simulink model "Gen_stAlone"  (R2018a)
settings: Solver=VariableStepAuto  StartTime=0.0  StopTime=20  MaxStep=1e-3  RelTol=1e-3
libraries: simulink x1
settings Model: Creator=cmparedes  LastModifiedBy=cmparedes

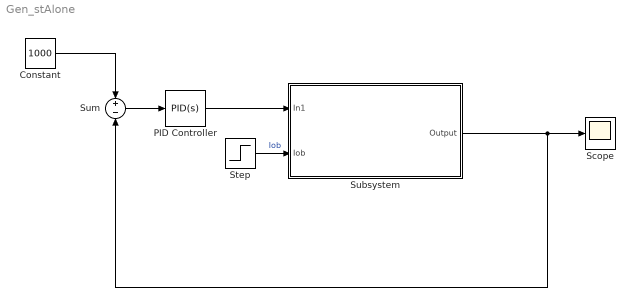
== system Gen_stAlone ==
  Constant : Constant  Value=1000
  PID Controller : simulink/Continuous/PID Controller  Controller=PID  TimeDomain=Continuous-time  SampleTime=-1  IntegratorMethod=Forward Euler  FilterMethod=Forward Euler  Form=Parallel  UseFilter=on  ControllerParametersSource=internal  P=1  I=10  D=0  N=100  InitialConditionSource=internal  InitialConditionForIntegrator=0  InitialConditionForFilter=0  ExternalReset=none  LimitOutput=off  UpperSaturationLimit=inf  LowerSaturationLimit=-inf  LinearizeAsGain=on  AntiWindupMode=none  Kb=1  TrackingMode=off  Kt=1  PParamMin=[]  PParamMax=[]  IParamMin=[]  IParamMax=[]  DParamMin=[]  DParamMax=[]  NParamMin=[]  NParamMax=[]  KbParamMin=[]  KbParamMax=[]  KtParamMin=[]  KtParamMax=[]  POutMin=[]  POutMax=[]  IOutMin=[]  IOutMax=[]  DOutMin=[]  DOutMax=[]  NOutMin=[]  NOutMax=[]  KbOutMin=[]  KbOutMax=[]  KtOutMin=[]  KtOutMax=[]  IntegratorOutMin=[]  IntegratorOutMax=[]  FilterOutMin=[]  FilterOutMax=[]  SumOutMin=[]  SumOutMax=[]  SumI1OutMin=[]  SumI1OutMax=[]  SumI2OutMin=[]  SumI2OutMax=[]  SumI3OutMin=[]  SumI3OutMax=[]  SumDOutMin=[]  SumDOutMax=[]  SaturationOutMin=[]  SaturationOutMax=[]  IntegratorContinuousStateAttributes=''  IntegratorStateMustResolveToSignalObject=off  IntegratorRTWStateStorageClass=Auto  FilterContinuousStateAttributes=''  FilterStateMustResolveToSignalObject=off  FilterRTWStateStorageClass=Auto  DifferentiatorICPrevScaledInput=0  DifferentiatorOutMin=[]  DifferentiatorOutMax=[]  FilterDiffOutCoefMin=[]  FilterDiffOutCoefMax=[]  SumDenOutMin=[]  SumDenOutMax=[]  SumNumOutMin=[]  SumNumOutMax=[]  ReciprocalOutMin=[]  ReciprocalOutMax=[]  DivideOutMin=[]  DivideOutMax=[]  TunerSelectOption=Transfer Function Based (PID Tuner App)
  Scope : Scope
  Step : Step  Time=10  Before=5  After=10  SampleTime=0
  Subsystem : Subsystem
  Sum : Sum  Inputs=+-
  wires:
  Step/1 -> Subsystem/2(Iob)  "Iob"
  Sum/1 -> PID Controller/1
  PID Controller/1 -> Subsystem/1(In1)
  Constant/1 -> Sum/1
  Subsystem/1(Output) -> Scope/1, Sum/2

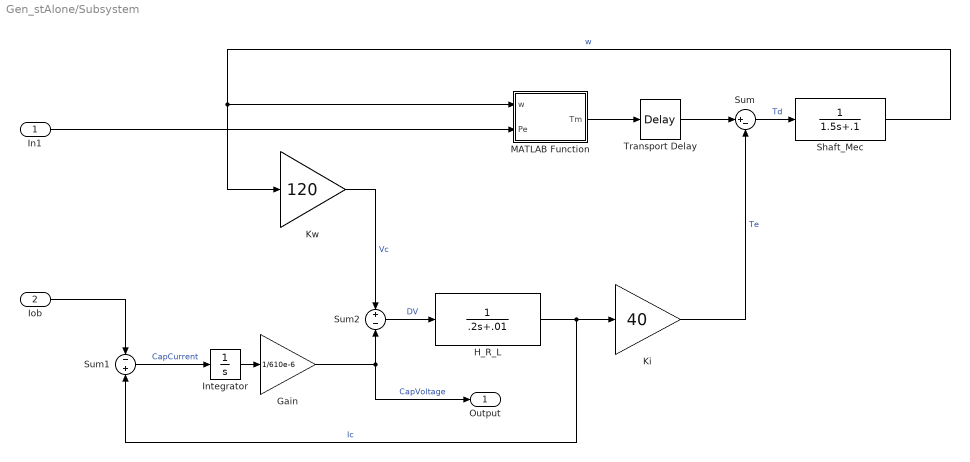
== system Gen_stAlone/Subsystem ==
  In1 : Inport
  Iob : Inport  Port=2
  Gain : Gain  Gain=1/610e-6
  H_R_L : TransferFcn  Denominator=[.2 .01]
  Integrator : Integrator
  Ki : Gain  Gain=40
  Kw : Gain  Gain=120
  MATLAB Function : MATLAB Function  TreatAsAtomicUnit=on
  Shaft_Mec : TransferFcn  Denominator=[1.5 .1]
  Sum : Sum  Inputs=|+-
  Sum1 : Sum  Inputs=-+
  Sum2 : Sum  Inputs=+-
  Transport Delay : TransportDelay  DelayTime=1e-6
  Output : Outport
  wires:
  Integrator/1 -> Gain/1
  Sum/1 -> Shaft_Mec/1  "Td"
  Gain/1 -> Output/1, Sum2/2  "CapVoltage"
  Transport Delay/1 -> Sum/1
  Kw/1 -> Sum2/1  "Vc"
  H_R_L/1 -> Sum1/2, Ki/1  "Ic"
  Sum1/1 -> Integrator/1  "CapCurrent"
  Shaft_Mec/1 -> Kw/1, MATLAB Function/1(w)  "w"
  MATLAB Function/1(Tm) -> Transport Delay/1
  Sum2/1 -> H_R_L/1  "DV"
  Ki/1 -> Sum/2  "Te"
  In1/1 -> MATLAB Function/2(Pe)
  Iob/1 -> Sum1/1

== matlab function Gen_stAlone/Subsystem/MATLAB Function ==
  data: w input; Pe input; Tm output
function Tm = fcn(w, Pe)

max_torq=30000;

if w>0
    Tm = Pe/w;
else
    Tm = max_torq;
end
